simulink model "TractorTrailer6DOF"  (R2024b)
settings: Solver=ode23tb  StartTime=0.0  StopTime=50  MaxStep=1.0  RelTol=1e-1  AbsTol=1e-5
model mask{initialTractorPosition=[0 0 0], initialTractorVelocity=[0 0 0], initialTractorOrientation=[0 0 0], initialTractorRotationRates=[0 0 0], initialTrailerPosition=[0 0 0], initialTrailerVelocity=[0 0 0], initialTrailerOrientation=[0 0 0], initialTrailerRotationRates=[0 0 0]}
  mask prompts: initialTractorPosition "Initial Tractor Position:"; initialTractorVelocity "Initial Tractor Velocity:"; initialTractorOrientation "Initial Tractor Orientation:"; initialTractorRotationRates "Initial Tractor Rotation Rates:"; initialTrailerPosition "Initial Trailer Position:"; initialTrailerVelocity "Initial Trailer Velocity:"; initialTrailerOrientation "Initial Trailer Orientation:"; initialTrailerRotationRates "Initial Trailer Rotation Rates:"
model workspace (MAT data in the model file):
  initialTractorOrientation = Simulink.Parameter
  initialTractorOrientation.Value = [0 0 0]
  initialTractorOrientation.Complexity = 'real'
  initialTractorOrientation.Dimensions = [1 3]
  initialTractorOrientation.DataType = 'auto'
  initialTractorPosition = Simulink.Parameter
  initialTractorPosition.Value = [0 0 0]
  initialTractorPosition.Complexity = 'real'
  initialTractorPosition.Dimensions = [1 3]
  initialTractorPosition.DataType = 'auto'
  initialTractorRotationRates = Simulink.Parameter
  initialTractorRotationRates.Value = [0 0 0]
  initialTractorRotationRates.Complexity = 'real'
  initialTractorRotationRates.Dimensions = [1 3]
  initialTractorRotationRates.DataType = 'auto'
  initialTractorVelocity = Simulink.Parameter
  initialTractorVelocity.Value = [0 0 0]
  initialTractorVelocity.Complexity = 'real'
  initialTractorVelocity.Dimensions = [1 3]
  initialTractorVelocity.DataType = 'auto'
  initialTrailerOrientation = Simulink.Parameter
  initialTrailerOrientation.Value = [0 0 0]
  initialTrailerOrientation.Complexity = 'real'
  initialTrailerOrientation.Dimensions = [1 3]
  initialTrailerOrientation.DataType = 'auto'
  initialTrailerPosition = Simulink.Parameter
  initialTrailerPosition.Value = [0 0 0]
  initialTrailerPosition.Complexity = 'real'
  initialTrailerPosition.Dimensions = [1 3]
  initialTrailerPosition.DataType = 'auto'
  initialTrailerRotationRates = Simulink.Parameter
  initialTrailerRotationRates.Value = [0 0 0]
  initialTrailerRotationRates.Complexity = 'real'
  initialTrailerRotationRates.Dimensions = [1 3]
  initialTrailerRotationRates.DataType = 'auto'
  initialTrailerVelocity = Simulink.Parameter
  initialTrailerVelocity.Value = [0 0 0]
  initialTrailerVelocity.Complexity = 'real'
  initialTrailerVelocity.Dimensions = [1 3]
  initialTrailerVelocity.DataType = 'auto'
undefined symbols (not defined in the file): hitch, tractor, trailer
libraries: autolibutils x7, sharedtransform x4, vehdynlibtire x4, vehdynlibeom x2, vehdynlibsuspension x2, vehdynlibtirecommon x2, simulink x1
(part 1 of 4)
settings Model: SimulationMode=accelerator  ParameterArgumentNames=initialTractorOrientation,initialTractorPosition,initialTractorRotationRates,initialTractorVelocity,initialTrailerOrientation,initialTrailerPosition,initialTrailerRotationRates,initialTrailerVelocity  Creator=The MathWorks, Inc.  LastModifiedBy=rsuresh
settings SolverCC: DateTimeAtSimulationTimeZero=[]  SolverJacobianMethodControl=FullPerturbation  ZeroCrossAlgorithm=Adaptive  DecoupledContinuousIntegration=on  MinimalZcImpactIntegration=on
settings DataIOCC: ReturnWorkspaceOutputsName=tp280c6351_3b58_4b1a_80b9_cf8454703752
settings OptimizationCC: ReuseModelBlockBuffer=off
settings DebuggingCC: IgnoredZcDiagnostic=none
settings RTWCC: GPUComputeCapability=3.5

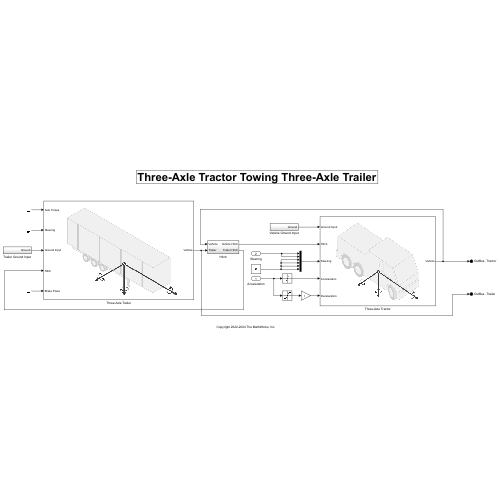
[thumbnail: Simulink's stored preview of the top-level diagram]
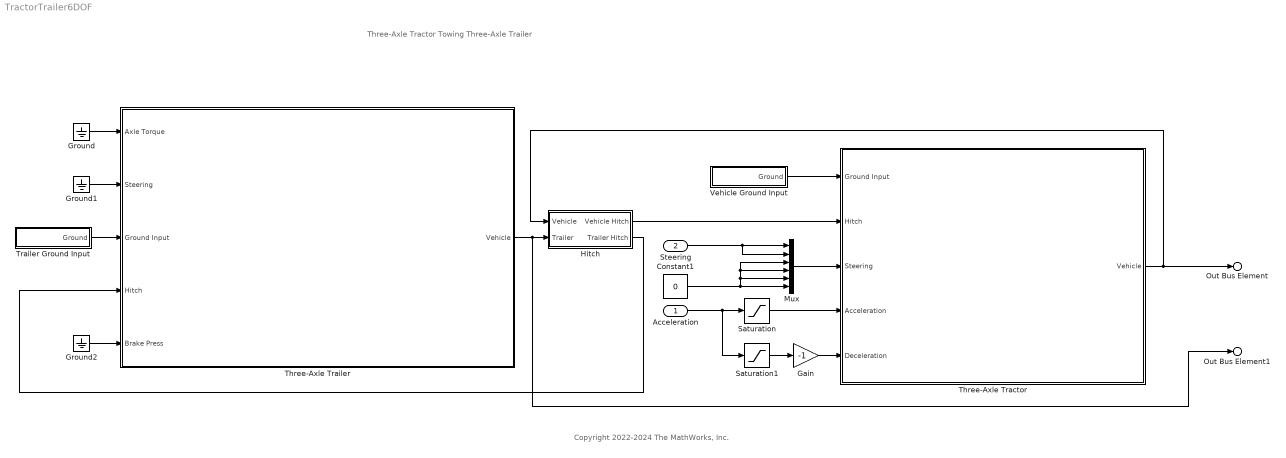
== system TractorTrailer6DOF ==
  note: Copyright 2022-2024 The MathWorks, Inc.
  note: Three-Axle Tractor Towing Three-Axle Trailer
  Acceleration : Inport
  Steering : Inport  Port=2
  Constant1 : Constant  Value=0
  Gain : Gain  Gain=-1
  Ground : Ground
  Ground1 : Ground
  Ground2 : Ground
  Hitch : Subsystem
  Mux : Mux  Inputs=6
  Saturation : Saturate  UpperLimit=3  LowerLimit=0  ZeroCross=off
  Saturation1 : Saturate  UpperLimit=0  LowerLimit=-9.8  ZeroCross=off
  Three-Axle Tractor : Subsystem
      mask Display: image('6dof3axletractor.png');
  Three-Axle Trailer : Subsystem
      mask Display: image('6dof3axletrailer.png');
  Trailer Ground Input : Subsystem  VariantControl=0
  Vehicle Ground Input : Subsystem  VariantControl=0
  Out Bus Element : Outport  PortName=OutBus  Element=Tractor
  Out Bus Element1 : Outport  PortName=OutBus  Element=Trailer
  wires:
  Ground2/1 -> Three-Axle Trailer/5(Brake Press)
  Gain/1 -> Three-Axle Tractor/5(Deceleration)
  Trailer Ground Input/1(Ground) -> Three-Axle Trailer/3(Ground Input)
  Ground/1 -> Three-Axle Trailer/1(Axle Torque)
  Vehicle Ground Input/1(Ground) -> Three-Axle Tractor/1(Ground Input)
  Ground1/1 -> Three-Axle Trailer/2(Steering)
  Hitch/2(Trailer Hitch) -> Three-Axle Trailer/4(Hitch)
  Mux/1 -> Three-Axle Tractor/3(Steering)
  Saturation1/1 -> Gain/1
  Saturation/1 -> Three-Axle Tractor/4(Acceleration)
  Hitch/1(Vehicle Hitch) -> Three-Axle Tractor/2(Hitch)
  Constant1/1 -> Mux/3, Mux/4, Mux/5, Mux/6
  Three-Axle Tractor/1(Vehicle) -> Out Bus Element/1, Hitch/1(Vehicle)
  Three-Axle Trailer/1(Vehicle) -> Out Bus Element1/1, Hitch/2(Trailer)
  Steering/1 -> Mux/2, Mux/1
  Acceleration/1 -> Saturation/1, Saturation1/1

== system TractorTrailer6DOF/Hitch ==
  Vehicle : Inport
  Trailer : Inport  Port=2
  Bus Selector : BusSelector  OutputSignals=Vehicle.InertFrm.Hitch.Disp.X,Vehicle.InertFrm.Hitch.Disp.Y,Vehicle.InertFrm.Hitch.Disp.Z,Vehicle.InertFrm.Hitch.Vel.Xdot,Vehicle.InertFrm.Hitch.Vel.Ydot,Vehicle.InertFrm.Hitch.Vel.Zdot,Vehicle.InertFrm.Cg.Ang.psi
  Bus Selector1 : BusSelector  OutputSignals=Vehicle.InertFrm.HitchF.Disp.X,Vehicle.InertFrm.HitchF.Disp.Y,Vehicle.InertFrm.HitchF.Disp.Z,Vehicle.InertFrm.HitchF.Vel.Xdot,Vehicle.InertFrm.HitchF.Vel.Ydot,Vehicle.InertFrm.HitchF.Vel.Zdot,Vehicle.InertFrm.Cg.Ang.psi
  Mux : Mux  Inputs=6
  Mux1 : Mux  Inputs=6
  Subsystem3 : Subsystem
  Vehicle Hitch : Outport
  Trailer Hitch : Outport  Port=2
  wires:
  Bus Selector1/5 -> Subsystem3/12(Trailer Ydot)  "<Ydot>"
  Subsystem3/5(Vehicle Mhy) -> Mux1/5
  Bus Selector/3 -> Subsystem3/3(Vehicle Z)  "<Z>"
  Subsystem3/12(Trailer Mhz) -> Mux/6
  Subsystem3/4(Vehicle Mhx) -> Mux1/4
  Subsystem3/10(Trailer Mhx) -> Mux/4
  Bus Selector/4 -> Subsystem3/4(Vehicle Xdot)  "<Xdot>"
  Subsystem3/11(Trailer Mhy) -> Mux/5
  Subsystem3/7(Trailer Fx) -> Mux/1
  Bus Selector1/1 -> Subsystem3/8(Trailer X)  "<X>"
  Bus Selector/5 -> Subsystem3/5(Vehicle Ydot)  "<Ydot>"
  Trailer/1 -> Bus Selector1/1
  Bus Selector1/4 -> Subsystem3/11(Trailer Xdot)  "<Xdot>"
  Subsystem3/6(Vehicle Mhz) -> Mux1/6
  Subsystem3/2(Vehicle Fy) -> Mux1/2
  Bus Selector/2 -> Subsystem3/2(Vehicle Y)  "<Y>"
  Bus Selector1/2 -> Subsystem3/9(Trailer Y)  "<Y>"
  Bus Selector1/6 -> Subsystem3/13(Trailer Zdot)  "<Zdot>"
  Subsystem3/1(Vehicle Fx) -> Mux1/1
  Bus Selector1/3 -> Subsystem3/10(Trailer Z)  "<Z>"
  Bus Selector/1 -> Subsystem3/1(Vehicle X)  "<X>"
  Subsystem3/8(Trailer Fy) -> Mux/2
  Bus Selector1/7 -> Subsystem3/14(Trailer psi)  "<psi>"
  Subsystem3/9(Trailer Fz) -> Mux/3
  Bus Selector/7 -> Subsystem3/7(Vehicle psi)  "<psi>"
  Mux/1 -> Trailer Hitch/1
  Bus Selector/6 -> Subsystem3/6(Vehicle Zdot)  "<Zdot>"
  Subsystem3/3(Vehicle Fz) -> Mux1/3
  Vehicle/1 -> Bus Selector/1
  Mux1/1 -> Vehicle Hitch/1

== system TractorTrailer6DOF/Three-Axle Tractor ==
  Ground Input : Inport
  Hitch : Inport  Port=2
  Steering : Inport  Port=3
  Acceleration : Inport  Port=4
  Deceleration : Inport  Port=5
  Brake System : Subsystem
  Brakes : BusCreator  Inputs=1
  Bus Creator : BusCreator  Inputs=4
  Bus Selector : BusSelector  OutputSignals=z,mu
  Subsystem1 : Subsystem
  Vehicle Body : Subsystem
  Vehicle Suspension : Subsystem
  Wheels and Tires : Subsystem
  Vehicle : Outport
  wires:
  Bus Selector/1 -> Wheels and Tires/4(Ground Input)  "<z>"
  Hitch/1 -> Vehicle Body/2(Hitch)
  Vehicle Suspension/1(Suspension) -> Wheels and Tires/1(Suspension), Bus Creator/2, Vehicle Body/1(Suspension)  "Suspension"
  Vehicle Body/1(Vehicle) -> Bus Creator/1, Vehicle Suspension/3(Vehicle), Brake System/2(Vehicle)  "Vehicle"
  Wheels and Tires/1(Wheels) -> Vehicle Suspension/2(Wheels), Bus Creator/3  "Wheels"
  Bus Selector/2 -> Wheels and Tires/5(Friction)  "<mu>"
  Steering/1 -> Vehicle Suspension/1(Steering)
  Ground Input/1 -> Bus Selector/1
  Bus Creator/1 -> Vehicle/1
  Brake System/1(Brake Press) -> Brakes/1, Wheels and Tires/3(Brake Press)  "Pressure"
  Deceleration/1 -> Brake System/1(Deceleration)
  Brakes/1 -> Bus Creator/4  "Brakes"
  Subsystem1/1(TAxles) -> Wheels and Tires/2(Axle Torque)
  Wheels and Tires/2(AxlPwr) -> [AxlPwr]
  Wheels and Tires/3(Omega) -> [Omega]
  Acceleration/1 -> Subsystem1/1(Acceleration)
  [AxlPwr] -> Subsystem1/2(AxlPwr)
  [Omega] -> Subsystem1/3(Omega)

== system TractorTrailer6DOF/Three-Axle Trailer ==
  Axle Torque : Inport
  Steering : Inport  Port=2
  Ground Input : Inport  Port=3
  Hitch : Inport  Port=4
  Brake Press : Inport  Port=5
  Brakes : BusCreator  Inputs=1
  Bus Creator : BusCreator  Inputs=4
  Bus Selector : BusSelector  OutputSignals=z,mu
  Trailer Suspension : Subsystem
  Vehicle Body : Subsystem
  Wheels and Tires : Subsystem
  Vehicle : Outport
  wires:
  Bus Creator/1 -> Vehicle/1
  Ground Input/1 -> Bus Selector/1
  Steering/1 -> Trailer Suspension/1(Steering)
  Axle Torque/1 -> Wheels and Tires/2(Axle Torque)
  Bus Selector/2 -> Wheels and Tires/5(Friction)  "<mu>"
  Wheels and Tires/1(Wheels) -> Trailer Suspension/2(Wheels), Bus Creator/3  "Wheels"
  Vehicle Body/1(Vehicle) -> Bus Creator/1, Trailer Suspension/3(Vehicle)  "Vehicle"
  Trailer Suspension/1(Suspension) -> Wheels and Tires/1(Suspension), Bus Creator/2, Vehicle Body/1(Suspension)  "Suspension"
  Hitch/1 -> Vehicle Body/2(Hitch)
  Bus Selector/1 -> Wheels and Tires/4(Ground Input)  "<z>"
  Brakes/1 -> Bus Creator/4  "Brakes"
  Brake Press/1 -> Wheels and Tires/3(Brake Press), Brakes/1  "Pressure"

== system TractorTrailer6DOF/Trailer Ground Input ==
  Bus Creator : BusCreator  Inputs=6
  Bus Creator2 : BusCreator  Inputs=6
  Bus Creator3 : BusCreator  Inputs=2
  Constant1 : Constant  Value=zeros(6,1)
  Demux : Demux  Outputs=6
  Demux1 : Demux  Outputs=6
  Friction : Constant  Value=ones(6,1).*1.0
  Signal Specification : SignalSpecification  Unit=m
  Signal Specification1 : SignalSpecification  Unit=1
  Ground : Outport  VectorParamsAs1DForOutWhenUnconnected=off
  wires:
  Constant1/1 -> Signal Specification/1
  Signal Specification/1 -> Demux/1
  Demux/6 -> Bus Creator/6  "G_RR_z"
  Demux/1 -> Bus Creator/1  "G_FL_z"
  Demux/5 -> Bus Creator/5  "G_RL_z"
  Demux/2 -> Bus Creator/2  "G_FR_z"
  Bus Creator/1 -> Bus Creator3/1  "z"
  Demux1/5 -> Bus Creator2/5  "mu_RL"
  Demux1/6 -> Bus Creator2/6  "mu_RR"
  Demux1/1 -> Bus Creator2/1  "mu_FL"
  Demux1/2 -> Bus Creator2/2  "mu_FR"
  Bus Creator2/1 -> Bus Creator3/2  "mu"
  Friction/1 -> Signal Specification1/1
  Signal Specification1/1 -> Demux1/1
  Bus Creator3/1 -> Ground/1
  Demux/3 -> Bus Creator/3  "G_ML_z"
  Demux/4 -> Bus Creator/4  "G_MR_z"
  Demux1/3 -> Bus Creator2/3  "mu_ML"
  Demux1/4 -> Bus Creator2/4  "mu_MR"

== system TractorTrailer6DOF/Vehicle Ground Input ==
  Bus Creator : BusCreator  Inputs=6
  Bus Creator2 : BusCreator  Inputs=6
  Bus Creator3 : BusCreator  Inputs=2
  Constant1 : Constant  Value=zeros(6,1)
  Demux : Demux  Outputs=6
  Demux1 : Demux  Outputs=6
  Friction : Constant  Value=ones(6,1).*1.0
  Signal Specification : SignalSpecification  Unit=m
  Signal Specification1 : SignalSpecification  Unit=1
  Ground : Outport  VectorParamsAs1DForOutWhenUnconnected=off
  wires:
  Demux1/4 -> Bus Creator2/4  "mu_MR"
  Demux1/3 -> Bus Creator2/3  "mu_ML"
  Demux/4 -> Bus Creator/4  "G_MR_z"
  Demux/3 -> Bus Creator/3  "G_ML_z"
  Bus Creator3/1 -> Ground/1
  Signal Specification1/1 -> Demux1/1
  Friction/1 -> Signal Specification1/1
  Bus Creator2/1 -> Bus Creator3/2  "mu"
  Demux1/2 -> Bus Creator2/2  "mu_FR"
  Demux1/1 -> Bus Creator2/1  "mu_FL"
  Demux1/6 -> Bus Creator2/6  "mu_RR"
  Demux1/5 -> Bus Creator2/5  "mu_RL"
  Bus Creator/1 -> Bus Creator3/1  "z"
  Demux/2 -> Bus Creator/2  "G_FR_z"
  Demux/5 -> Bus Creator/5  "G_RL_z"
  Demux/1 -> Bus Creator/1  "G_FL_z"
  Demux/6 -> Bus Creator/6  "G_RR_z"
  Signal Specification/1 -> Demux/1
  Constant1/1 -> Signal Specification/1

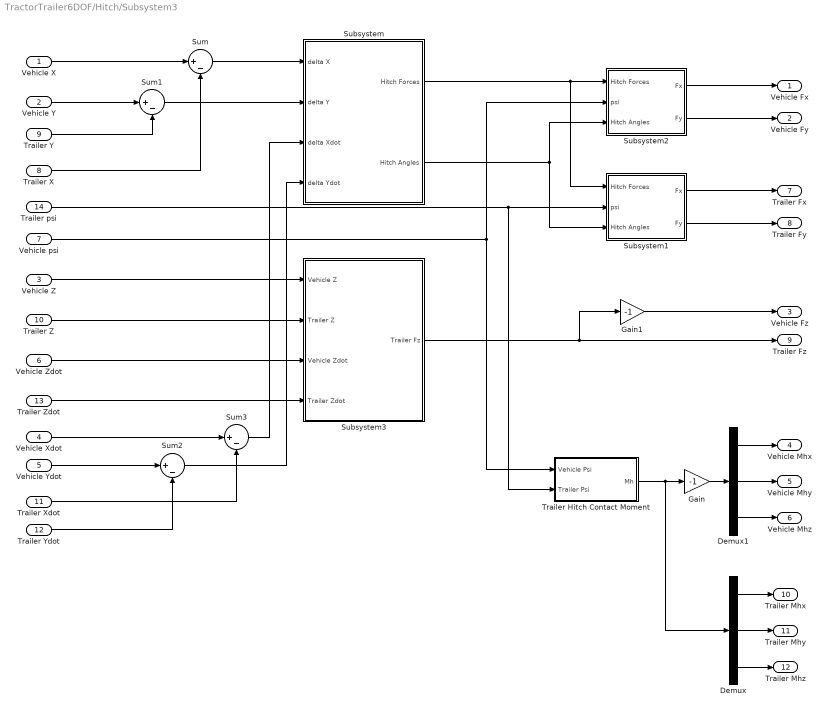
== system TractorTrailer6DOF/Hitch/Subsystem3 ==
  Vehicle X : Inport
  Vehicle Y : Inport  Port=2
  Vehicle Z : Inport  Port=3
  Vehicle Xdot : Inport  Port=4
  Vehicle Ydot : Inport  Port=5
  Vehicle Zdot : Inport  Port=6
  Vehicle psi : Inport  Port=7
  Trailer X : Inport  Port=8
  Trailer Y : Inport  Port=9
  Trailer Z : Inport  Port=10
  Trailer Xdot : Inport  Port=11
  Trailer Ydot : Inport  Port=12
  Trailer Zdot : Inport  Port=13
  Trailer psi : Inport  Port=14
  Demux : Demux  Outputs=3
  Demux1 : Demux  Outputs=3
  Gain : Gain  Gain=-1
  Gain1 : Gain  Gain=-1
  Subsystem : Subsystem
  Subsystem1 : Subsystem
  Subsystem2 : Subsystem
  Subsystem3 : Subsystem
  Sum{,1..3} (4 alike) : Sum  Inputs=|+-
  Trailer Hitch Contact Moment : Subsystem
  Vehicle Fx : Outport
  Vehicle Fy : Outport  Port=2
  Vehicle Fz : Outport  Port=3
  Vehicle Mhx : Outport  Port=4
  Vehicle Mhy : Outport  Port=5
  Vehicle Mhz : Outport  Port=6
  Trailer Fx : Outport  Port=7
  Trailer Fy : Outport  Port=8
  Trailer Fz : Outport  Port=9
  Trailer Mhx : Outport  Port=10
  Trailer Mhy : Outport  Port=11
  Trailer Mhz : Outport  Port=12
  wires:
  Subsystem/1(Hitch Forces) -> Subsystem2/1(Hitch Forces), Subsystem1/1(Hitch Forces)
  Sum/1 -> Subsystem/1(delta X)
  Sum1/1 -> Subsystem/2(delta Y)
  Vehicle X/1 -> Sum/1
  Trailer Y/1 -> Sum1/2
  Trailer X/1 -> Sum/2
  Vehicle Y/1 -> Sum1/1
  Trailer psi/1 -> Trailer Hitch Contact Moment/2(Trailer Psi), Subsystem1/2(psi)
  Vehicle psi/1 -> Subsystem2/2(psi), Trailer Hitch Contact Moment/1(Vehicle Psi)
  Subsystem/2(Hitch Angles) -> Subsystem2/3(Hitch Angles), Subsystem1/3(Hitch Angles)
  Subsystem3/1(Trailer Fz) -> Gain1/1, Trailer Fz/1
  Subsystem2/1(Fx) -> Vehicle Fx/1
  Subsystem2/2(Fy) -> Vehicle Fy/1
  Subsystem1/1(Fx) -> Trailer Fx/1
  Subsystem1/2(Fy) -> Trailer Fy/1
  Vehicle Z/1 -> Subsystem3/1(Vehicle Z)
  Trailer Z/1 -> Subsystem3/2(Trailer Z)
  Gain1/1 -> Vehicle Fz/1
  Vehicle Zdot/1 -> Subsystem3/3(Vehicle Zdot)
  Trailer Zdot/1 -> Subsystem3/4(Trailer Zdot)
  Trailer Ydot/1 -> Sum2/2
  Vehicle Xdot/1 -> Sum3/1
  Vehicle Ydot/1 -> Sum2/1
  Trailer Xdot/1 -> Sum3/2
  Sum2/1 -> Subsystem/4(delta Ydot)
  Sum3/1 -> Subsystem/3(delta Xdot)
  Demux/1 -> Trailer Mhx/1
  Demux1/3 -> Vehicle Mhz/1
  Demux/2 -> Trailer Mhy/1
  Demux1/2 -> Vehicle Mhy/1
  Trailer Hitch Contact Moment/1(Mh) -> Demux/1, Gain/1
  Demux1/1 -> Vehicle Mhx/1
  Demux/3 -> Trailer Mhz/1
  Gain/1 -> Demux1/1

== system TractorTrailer6DOF/Three-Axle Tractor/Brake System ==
  Deceleration : Inport
  Vehicle : Inport  Port=2
  Bus Selector : BusSelector  OutputSignals=BdyFrm.Cg.Vel.xdot
  Constant : Constant  Value=0
  Hydraulics : autolibutils/Cont LPF  wc=30*pi*2  AbsoluteTolerance=auto  aMode=2
  Mux : Mux  Inputs=6
  Pressure : Gain  Gain=2e5
  Pressure1 : Gain  Gain=1e6
  Saturation1 : Saturate  UpperLimit=inf  LowerLimit=0  ZeroCross=off
  Signal Specification : SignalSpecification  Unit=Pa
  Switch : Switch  Criteria=u2 > Threshold  Threshold=0.1  ZeroCross=off  SaturateOnIntegerOverflow=off  InputSameDT=off
  Brake Press : Outport  PortDimensions=6  VectorParamsAs1DForOutWhenUnconnected=off
  wires:
  Signal Specification/1 -> Brake Press/1
  Mux/1 -> Signal Specification/1
  Saturation1/1 -> Hydraulics/1
  Hydraulics/1 -> Pressure1/1, Pressure/1
  Pressure/1 -> Mux/2, Mux/1
  Vehicle/1 -> Bus Selector/1
  Switch/1 -> Saturation1/1
  Deceleration/1 -> Switch/1
  Bus Selector/1 -> Switch/2  "<xdot>"
  Constant/1 -> Switch/3
  Pressure1/1 -> Mux/6, Mux/4, Mux/3, Mux/5

== system TractorTrailer6DOF/Three-Axle Tractor/Subsystem1 ==
  Acceleration : Inport
  AxlPwr : Inport  Port=2
  Omega : Inport  Port=3
  Constant : Constant
  Driveline : Subsystem  Variant=on  VariantControlMode=label  VariantControl=Variant1  LabelModeActiveChoice=0
  Powertrain : Subsystem
  TAxles : Outport
  wires:
  Powertrain/1(AxlTrq) -> Driveline/1(TPowertrain)
  Acceleration/1 -> Powertrain/1(Acc)
  Omega/1 -> Powertrain/3(Omega)
  AxlPwr/1 -> Powertrain/2(AxlPwr)
  Driveline/1(TAxles) -> TAxles/1
  Constant/1 -> Driveline/2(Gear)

== system TractorTrailer6DOF/Three-Axle Tractor/Vehicle Body ==
  Suspension : Inport
  Hitch : Inport  Port=2
  Bus Selector3 : BusSelector  OutputSignals=Veh.F,Veh.M
  Constant : Constant  Value=zeros(3,1)
  Ground : Ground
  Ground1 : Ground
  Selector6 : Selector  InputPortWidth=6  IndexOptions=Index vector (dialog)  Indices=[1 2 3]  OutputSizes=1
  Selector7 : Selector  InputPortWidth=6  IndexOptions=Index vector (dialog)  Indices=[4 5 6]  OutputSizes=1
  Terminator{6..11} (6 alike) : Terminator
  Vehicle Body 6DOF Three Axles : vehdynlibeom/Vehicle Body 6DOF Three Axles  extPos=on  extVel=on  extEuler=on  extRotRate=on  htchFMode=on  htchMMode=on  m=tractor.Mass  a=tractor.FrontAxlePositionfromCG  b=tractor.MiddleAxlePositionFromCG  c=tractor.RearAxlePositionfromCG  d=0  h=tractor.HeightCG  dh=tractor.HitchDistance  hl=0  hh=tractor.HitchHeight  Xe_o=initialTractorPosition  xbdot_o=initialTractorVelocity  eul_o=initialTractorOrientation  p_o=initialTractorRotationRates  Iveh=[tractor.RollMomentInertia 0 0; 0 tractor.PitchMomentInertia 0; 0 0 tractor.YawMomentInertia]  w=tractor.TrackWidth.*[1 1 1]  z1m=0  z1R=[-.25,.125,.15]  z1I=[1.4,-.2,.1;-.2,1.4,.1;.1,.1,2.25].*0  z2m=0  z2R=[1.4,0,.8]  z2I=[1.4,-.2,.1;-.2,1.4,.1;.1,.1,2.25].*0  z3m=0  z3R=[.75,-.5,.4]  z3I=[5,-.1,-2;-2,9,.1;-.1,.1,6].*0  z4m=0  z4R=[.75,.5,.4]  z4I=[5,-.1,-2;-2,9,.1;-.1,.1,6].*0  z5m=0  z5R=[1.25,-.5,.4]  z5I=[5,-.1,-2;-2,9,.1;-.1,.1,6].*0  z6m=0  z6R=[1.25,-.5,.4]  z6I=[5,-.1,-2;-2,9,.1;-.1,.1,6].*0  z7m=0  z7R=[2,0,.25]  z7I=[1.4,-.2,.1;-.2,1.4,.1;.1,.1,2.25].*0  Af=tractor.FrontalArea  Cd=.3  Cl=.1  Cpm=.1  beta_w=[0:0.01:0.3]  Cs=[0:0.03:0.9]  Cym=[0:0.01:0.3]  Pabs=101325  extTamb=off  Tair=273  g=9.81  xdot_tol=.1  longOff=0  latOff=0  vertOff=0.0112  wrapAng=off  aMode=2
  Vehicle : Outport
  wires:
  Suspension/1 -> Bus Selector3/1
  Selector6/1 -> Vehicle Body 6DOF Three Axles/5
  Vehicle Body 6DOF Three Axles/2 -> Terminator6/1
  Hitch/1 -> Selector7/1, Selector6/1
  Vehicle Body 6DOF Three Axles/4 -> Terminator8/1
  Ground/1 -> Vehicle Body 6DOF Three Axles/3
  Vehicle Body 6DOF Three Axles/6 -> Terminator10/1
  Selector7/1 -> Vehicle Body 6DOF Three Axles/6
  Constant/1 -> Vehicle Body 6DOF Three Axles/7
  Vehicle Body 6DOF Three Axles/1 -> Vehicle/1
  Vehicle Body 6DOF Three Axles/3 -> Terminator7/1
  Bus Selector3/2 -> Vehicle Body 6DOF Three Axles/2  "<M>"
  Bus Selector3/1 -> Vehicle Body 6DOF Three Axles/1  "<F>"
  Vehicle Body 6DOF Three Axles/7 -> Terminator11/1
  Ground1/1 -> Vehicle Body 6DOF Three Axles/4
  Vehicle Body 6DOF Three Axles/5 -> Terminator9/1

== system TractorTrailer6DOF/Three-Axle Tractor/Vehicle Suspension ==
  Steering : Inport
  Wheels : Inport  Port=2
  Vehicle : Inport  Port=3
  Bus Creator1 : BusCreator  Inputs=5
  Bus Creator2 : BusCreator  Inputs=2
  Bus Creator3 : BusCreator  Inputs=2
  Bus Creator4 : BusCreator  Inputs=6
  Bus Selector : BusSelector  OutputSignals=z,Re,zdot,Fx,Fy,M
  Bus Selector1 : BusSelector  OutputSignals=P,V
  Selector1 : Selector  NumberOfDimensions=2  InputPortWidth=3  IndexOptions=Index vector (dialog),Select all  Indices=1,1  OutputSizes=1,1
  Selector2 : Selector  NumberOfDimensions=2  InputPortWidth=3  IndexOptions=Index vector (dialog),Select all  Indices=2,1  OutputSizes=1,1
  Solid Axle Suspension - Coil Spring : vehdynlibsuspension/Solid Axle Suspension - Coil Spring  NumAxl=3  NumWhlsByAxl=[2 2 2]  StrgEnByAxl=[1 1 1]  WhlNumVec="[1  2  1  2  1  2]"  AxleNumVec="[1  1  2  2  3  3]"  SuspTypesByAxle="[1  1  1]"  SuspImage=suspsacoil.png  AxlIxx=450  AxlM=500  TrackCoords=[zeros(1,6);tractor.TrackWidth*[1 -1 1 -1 1 -1]/2;zeros(1,6)]  SuspCoords=[zeros(1,6);tractor.TrackWidth*[1 -1 1 -1 1 -1]/2;zeros(1,6)]  KzWhlAxl=kzWhlAxl  F0zWhlAxl=f0zWhlAxl  CzWhlAxl=czWhlAxl  IdealSuspEn=on  IdealSuspAxles="[1  2  3]"  Kz=tractor.Kz  F0z=tractor.F0z  Cz=tractor.Cz  Hmax=hMax  Toe=0  RollStrgSlp=0  ToeStrgSlp=0  Caster=0  CasterHslp=0  CasterStrgSlp=0  Camber=0  CamberHslp=0  CamberStrgSlp=0  StrgHgtSlp=0.1432  MappedSuspEn=off  MappedSuspAxles="[1  2]"  f_susp_axl_bp=[1 2]  f_susp_dz_bp=[-0.15 -0.14 -0.13 -0.12 -0.11 -0.10 -0.09 -0.08 -0.07 -0.06 -0.05 -0.04 -0.03 -0.02 -0.01 0.00 0.01 0.02 0.03 0.04 0.05 0.06 0.07 0.08 0.09 0.10 0.11 0.12 0.13 0.14 0.15]  f_susp_dzdot_bp=[-0.15 -0.14 -0.13 -0.12 -0.11 -0.10 -0.09 -0.08 -0.07 -0.06 -0.05 -0.04 -0.03 -0.02 -0.01 0.00 0.01 0.02 0.03 0.04 0.05 0.06 0.07 0.08 0.09 0.10 0.11 0.12 0.13 0.14 0.15]  f_susp_fmz=zeros(31,31,61,2,4)  f_susp_geom=zeros(31,61,2,3)  f_susp_strgdelta_bp=[-30,-29,-28,-27,-26,-25,-24,-23,-22,-21,-20,-19,-18,-17,-16,-15,-14,-13,-12,-11,-10,-9,-8,-7,-6,-5,-4,-3,-2,-1,0,1,2,3,4,5,6,7,8,9,10,11,12,13,14,15,16,17,18,19,20,21,22,23,24,25,26,27,28,29,30]
  Steer Rate Adapter : Subsystem
  Steering Adapter : Subsystem
  Terminator1 : Terminator
  Terminator6 : Terminator
  Vehicle Adapter : Subsystem
  Wheel  Adapter : Subsystem
  Suspension : Outport
  wires:
  Wheel  Adapter/6(Re) -> Bus Creator4/6
  Bus Selector1/1 -> Solid Axle Suspension - Coil Spring/7  "<P>"
  Bus Selector/6 -> Solid Axle Suspension - Coil Spring/6  "<M>"
  Bus Selector/1 -> Solid Axle Suspension - Coil Spring/1  "<z>"
  Bus Selector/5 -> Solid Axle Suspension - Coil Spring/5  "<Fy>"
  Wheel  Adapter/1(WhlFx) -> Bus Creator4/1  "Fx"
  Bus Selector/4 -> Solid Axle Suspension - Coil Spring/4  "<Fx>"
  Wheel  Adapter/4(zdot) -> Bus Creator4/4
  Wheel  Adapter/2(WhlFy) -> Bus Creator4/2  "Fy"
  Solid Axle Suspension - Coil Spring/1 -> Terminator6/1
  Vehicle Adapter/1(VehSusp) -> Bus Selector1/1
  Bus Creator4/1 -> Bus Selector/1
  Bus Selector1/2 -> Solid Axle Suspension - Coil Spring/8  "<V>"
  Steering/1 -> Steering Adapter/1(Steer)
  Bus Selector/3 -> Solid Axle Suspension - Coil Spring/3  "<zdot>"
  Wheel  Adapter/3(z) -> Bus Creator4/3
  Wheel  Adapter/5(M) -> Bus Creator4/5
  Bus Selector/2 -> Solid Axle Suspension - Coil Spring/2  "<Re>"
  Vehicle Adapter/2(VehVBody) -> Selector1/1, Selector2/1
  Wheels/1 -> Wheel  Adapter/1(Wheels)
  Steering Adapter/1(StrgAng) -> Solid Axle Suspension - Coil Spring/9
  Vehicle/1 -> Vehicle Adapter/1(Veh), Steer Rate Adapter/1(Veh)
  Bus Creator3/1 -> Suspension/1
  Selector2/1 -> Bus Creator1/3  "ydot"
  Bus Creator2/1 -> Bus Creator3/1  "Veh"
  Solid Axle Suspension - Coil Spring/3 -> Bus Creator2/2  "M"
  Selector1/1 -> Bus Creator1/2  "xdot"
  Solid Axle Suspension - Coil Spring/6 -> Bus Creator1/4  "Ang"
  Bus Creator1/1 -> Bus Creator3/2  "Whl"
  Steer Rate Adapter/1(AngVel) -> Bus Creator1/5
  Solid Axle Suspension - Coil Spring/2 -> Bus Creator2/1  "F"
  Solid Axle Suspension - Coil Spring/4 -> Bus Creator1/1  "F"
  Solid Axle Suspension - Coil Spring/5 -> Terminator1/1

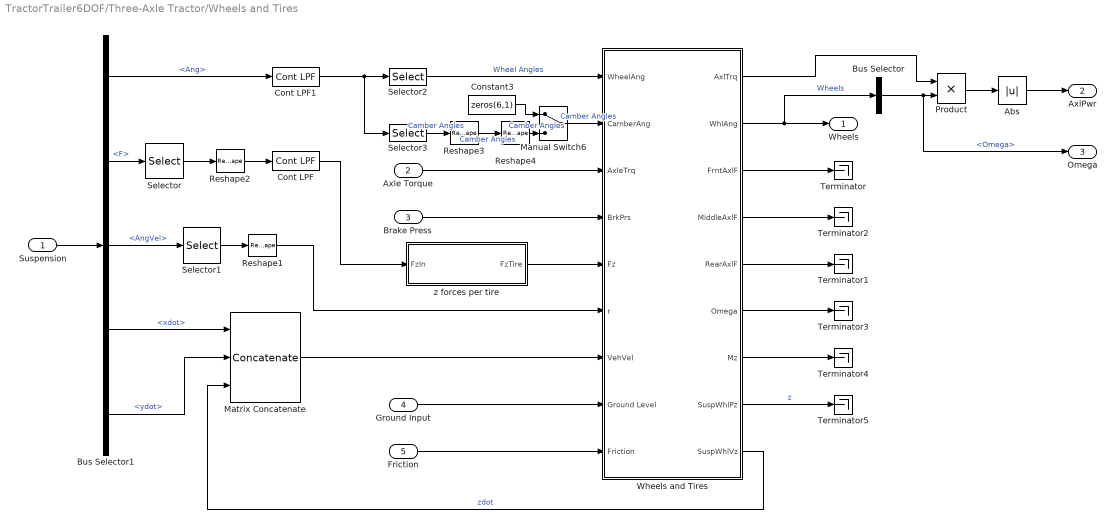
== system TractorTrailer6DOF/Three-Axle Tractor/Wheels and Tires ==
  Suspension : Inport
  Axle Torque : Inport  Port=2
  Brake Press : Inport  Port=3  Unit=Pa
  Ground Input : Inport  Port=4
  Friction : Inport  Port=5
  Abs : Abs  SaturateOnIntegerOverflow=off
  Bus Selector : BusSelector  OutputSignals=TireFrame.Omega
  Bus Selector1 : BusSelector  OutputSignals=Whl.Ang,Whl.F,Whl.AngVel,Whl.xdot,Whl.ydot
  Constant3 : Constant  Value=zeros(6,1)
  Cont LPF : autolibutils/Cont LPF  wc=100*2*pi  AbsoluteTolerance=auto  aMode=2
  Cont LPF1 : autolibutils/Cont LPF  wc=100*2*pi  AbsoluteTolerance=auto  aMode=2
  Manual Switch6 : ManualSwitch
  Matrix Concatenate : Concatenate  NumInputs=3  Mode=Multidimensional array
  Product : Product
  Reshape1 : Reshape
  Reshape2 : Reshape
  Reshape3 : Reshape  OutputDimensionality=Column vector (2-D)
  Reshape4 : Reshape
  Selector : Selector  NumberOfDimensions=2  InputPortWidth=3  IndexOptions=Index vector (dialog),Select all  Indices=[3],1  OutputSizes=1,1
  Selector1 : Selector  NumberOfDimensions=2  InputPortWidth=1  IndexOptions=Index vector (dialog),Select all  Indices=[3],1  OutputSizes=1,1
  Selector2 : Selector  NumberOfDimensions=2  InputPortWidth=3  IndexOptions=Index vector (dialog),Select all  Indices=3,1  OutputSizes=1,1
  Selector3 : Selector  NumberOfDimensions=2  InputPortWidth=3  IndexOptions=Index vector (dialog),Select all  Indices=1,1  OutputSizes=1,1
  Terminator{,1..5} (6 alike) : Terminator
  Wheels and Tires : Subsystem  VariantControl=0
  z forces per tire : Subsystem
  Wheels : Outport  VectorParamsAs1DForOutWhenUnconnected=off
  AxlPwr : Outport  Port=2
  Omega : Outport  Port=3
  wires:
  Wheels and Tires/2(WhlAng) -> Bus Selector/1, Wheels/1  "Wheels"
  Bus Selector1/2 -> Selector/1  "<F>"
  Wheels and Tires/3(FrntAxlF) -> Terminator/1
  Wheels and Tires/5(RearAxlF) -> Terminator1/1
  Wheels and Tires/6(Omega) -> Terminator3/1
  Wheels and Tires/7(Mz) -> Terminator4/1
  Selector1/1 -> Reshape1/1
  Matrix Concatenate/1 -> Wheels and Tires/7(VehVel)
  Axle Torque/1 -> Wheels and Tires/3(AxleTrq)
  Selector2/1 -> Wheels and Tires/1(WheelAng)  "Wheel Angles"
  Constant3/1 -> Manual Switch6/1
  Manual Switch6/1 -> Wheels and Tires/2(CamberAng)  "Camber Angles"
  Selector/1 -> Reshape2/1
  z forces per tire/1(FzTire) -> Wheels and Tires/5(Fz)
  Ground Input/1 -> Wheels and Tires/8(Ground Level)
  Wheels and Tires/9(SuspWhlVz) -> Matrix Concatenate/3  "zdot"
  Bus Selector1/1 -> Cont LPF1/1  "<Ang>"
  Selector3/1 -> Reshape3/1  "Camber Angles"
  Suspension/1 -> Bus Selector1/1
  Bus Selector1/4 -> Matrix Concatenate/1  "<xdot>"
  Bus Selector1/5 -> Matrix Concatenate/2  "<ydot>"
  Wheels and Tires/8(SuspWhlPz) -> Terminator5/1  "z"
  Reshape2/1 -> Cont LPF/1
  Bus Selector1/3 -> Selector1/1  "<AngVel>"
  Reshape1/1 -> Wheels and Tires/6(r)
  Brake Press/1 -> Wheels and Tires/4(BrkPrs)
  Friction/1 -> Wheels and Tires/9(Friction)
  Cont LPF1/1 -> Selector3/1, Selector2/1
  Wheels and Tires/4(MiddleAxlF) -> Terminator2/1
  Reshape3/1 -> Reshape4/1  "Camber Angles"
  Reshape4/1 -> Manual Switch6/2  "Camber Angles"
  Cont LPF/1 -> z forces per tire/1(FzIn)
  Bus Selector/1 -> Omega/1, Product/2  "<Omega>"
  Wheels and Tires/1(AxlTrq) -> Product/1
  Product/1 -> Abs/1
  Abs/1 -> AxlPwr/1

== system TractorTrailer6DOF/Three-Axle Trailer/Trailer Suspension ==
  Steering : Inport
  Wheels : Inport  Port=2
  Vehicle : Inport  Port=3
  Bus Creator1 : BusCreator  Inputs=5
  Bus Creator2 : BusCreator  Inputs=2
  Bus Creator3 : BusCreator  Inputs=2
  Bus Creator4 : BusCreator  Inputs=6
  Bus Selector : BusSelector  OutputSignals=z,Re,zdot,Fx,Fy,M
  Bus Selector1 : BusSelector  OutputSignals=P,V
  Selector1 : Selector  NumberOfDimensions=2  InputPortWidth=3  IndexOptions=Index vector (dialog),Select all  Indices=1,1  OutputSizes=1,1
  Selector2 : Selector  NumberOfDimensions=2  InputPortWidth=3  IndexOptions=Index vector (dialog),Select all  Indices=2,1  OutputSizes=1,1
  Solid Axle Suspension - Coil Spring : vehdynlibsuspension/Solid Axle Suspension - Coil Spring  NumAxl=3  NumWhlsByAxl=[2 2 2]  StrgEnByAxl=[1 1 1]  WhlNumVec="[1  2  1  2  1  2]"  AxleNumVec="[1  1  2  2  3  3]"  SuspTypesByAxle="[1  1  1]"  SuspImage=suspsacoil.png  AxlIxx=450  AxlM=500  TrackCoords=[zeros(1,6);trailer.TrackWidth*[1 -1 1 -1 1 -1]/2;zeros(1,6)]  SuspCoords=[zeros(1,6);trailer.TrackWidth*[1 -1 1 -1 1 -1]/2;zeros(1,6)]  KzWhlAxl=kzWhlAxl  F0zWhlAxl=f0zWhlAxl  CzWhlAxl=czWhlAxl  IdealSuspEn=on  IdealSuspAxles="[1  2  3]"  Kz=trailer.Kz  F0z=trailer.F0z  Cz=trailer.Cz(1)  Hmax=hMax  Toe=0  RollStrgSlp=0  ToeStrgSlp=0  Caster=0  CasterHslp=0  CasterStrgSlp=0  Camber=0  CamberHslp=0  CamberStrgSlp=0  StrgHgtSlp=0.1432  MappedSuspEn=off  MappedSuspAxles="[1  2]"  f_susp_axl_bp=[1 2]  f_susp_dz_bp=[-0.15 -0.14 -0.13 -0.12 -0.11 -0.10 -0.09 -0.08 -0.07 -0.06 -0.05 -0.04 -0.03 -0.02 -0.01 0.00 0.01 0.02 0.03 0.04 0.05 0.06 0.07 0.08 0.09 0.10 0.11 0.12 0.13 0.14 0.15]  f_susp_dzdot_bp=[-0.15 -0.14 -0.13 -0.12 -0.11 -0.10 -0.09 -0.08 -0.07 -0.06 -0.05 -0.04 -0.03 -0.02 -0.01 0.00 0.01 0.02 0.03 0.04 0.05 0.06 0.07 0.08 0.09 0.10 0.11 0.12 0.13 0.14 0.15]  f_susp_fmz=zeros(31,31,61,2,4)  f_susp_geom=zeros(31,61,2,3)  f_susp_strgdelta_bp=[-30,-29,-28,-27,-26,-25,-24,-23,-22,-21,-20,-19,-18,-17,-16,-15,-14,-13,-12,-11,-10,-9,-8,-7,-6,-5,-4,-3,-2,-1,0,1,2,3,4,5,6,7,8,9,10,11,12,13,14,15,16,17,18,19,20,21,22,23,24,25,26,27,28,29,30]
  Steer Rate Adapter : Subsystem
  Steering Adapter : Subsystem
  Terminator1 : Terminator
  Terminator6 : Terminator
  Vehicle Adapter : Subsystem
  Wheel  Adapter : Subsystem
  Suspension : Outport
  wires:
  Steer Rate Adapter/1(AngVel) -> Bus Creator1/5
  Bus Creator1/1 -> Bus Creator3/2  "Whl"
  Solid Axle Suspension - Coil Spring/6 -> Bus Creator1/4  "Ang"
  Selector1/1 -> Bus Creator1/2  "xdot"
  Solid Axle Suspension - Coil Spring/3 -> Bus Creator2/2  "M"
  Bus Creator2/1 -> Bus Creator3/1  "Veh"
  Selector2/1 -> Bus Creator1/3  "ydot"
  Bus Creator3/1 -> Suspension/1
  Vehicle/1 -> Steer Rate Adapter/1(Veh), Vehicle Adapter/1(Veh)
  Steering Adapter/1(StrgAng) -> Solid Axle Suspension - Coil Spring/9
  Wheels/1 -> Wheel  Adapter/1(Wheels)
  Vehicle Adapter/1(VehVBody) -> Selector1/1, Selector2/1
  Bus Selector/2 -> Solid Axle Suspension - Coil Spring/2  "<Re>"
  Wheel  Adapter/5(M) -> Bus Creator4/5
  Wheel  Adapter/3(z) -> Bus Creator4/3
  Bus Selector/3 -> Solid Axle Suspension - Coil Spring/3  "<zdot>"
  Steering/1 -> Steering Adapter/1(Steer)
  Bus Selector1/2 -> Solid Axle Suspension - Coil Spring/8  "<V>"
  Bus Creator4/1 -> Bus Selector/1
  Solid Axle Suspension - Coil Spring/1 -> Terminator6/1
  Wheel  Adapter/2(WhlFy) -> Bus Creator4/2  "Fy"
  Wheel  Adapter/4(zdot) -> Bus Creator4/4
  Bus Selector/4 -> Solid Axle Suspension - Coil Spring/4  "<Fx>"
  Wheel  Adapter/1(WhlFx) -> Bus Creator4/1  "Fx"
  Bus Selector/5 -> Solid Axle Suspension - Coil Spring/5  "<Fy>"
  Bus Selector/1 -> Solid Axle Suspension - Coil Spring/1  "<z>"
  Bus Selector/6 -> Solid Axle Suspension - Coil Spring/6  "<M>"
  Bus Selector1/1 -> Solid Axle Suspension - Coil Spring/7  "<P>"
  Wheel  Adapter/6(Re) -> Bus Creator4/6
  Solid Axle Suspension - Coil Spring/2 -> Bus Creator2/1  "F"
  Solid Axle Suspension - Coil Spring/4 -> Bus Creator1/1  "F"
  Solid Axle Suspension - Coil Spring/5 -> Terminator1/1
  Vehicle Adapter/2(VehSusp) -> Bus Selector1/1

== system TractorTrailer6DOF/Three-Axle Trailer/Vehicle Body ==
  Suspension : Inport
  Hitch : Inport  Port=2
  Bus Selector3 : BusSelector  OutputSignals=Veh.F,Veh.M
  Constant1 : Constant  Value=zeros(3,1)
  Ground : Ground
  Ground1 : Ground
  Selector6 : Selector  InputPortWidth=6  IndexOptions=Index vector (dialog)  Indices=[1 2 3]  OutputSizes=1
  Selector7 : Selector  InputPortWidth=6  IndexOptions=Index vector (dialog)  Indices=[4 5 6]  OutputSizes=1
  Terminator{,1..5} (6 alike) : Terminator
  Trailer Body 6DOF : vehdynlibeom/Trailer Body 6DOF  axleMode=3  extPos=on  extVel=on  extEuler=on  extRotRate=on  htchFMode_f=on  htchMMode_f=on  htchFMode_r=off  htchMMode_r=off  m=trailer.Mass  a=trailer.FrontAxlePositionfromCG  b=trailer.MiddleAxlePositionFromCG  c=trailer.RearAxlePositionfromCG  d=0  h=trailer.HeightCG  dh_f=trailer.HitchDistance  hl_f=0  hh_f=trailer.HitchHeight  dh_r=1  hl_r=0  hh_r=0.1  Xe_o=initialTrailerPosition  xbdot_o=initialTrailerVelocity  eul_o=initialTrailerOrientation  p_o=initialTrailerRotationRates  Iveh=[trailer.RollMomentInertia 0 0; 0 trailer.PitchMomentInertia 0; 0 0 trailer.YawMomentInertia]  w_f=trailer.TrackWidth  w_m=trailer.TrackWidth  w_r=trailer.TrackWidth  z1m=0  z1R=[-.25,.125,.15]  z1I=[1.4,-.2,.1;-.2,1.4,.1;.1,.1,2.25].*0  z2m=0  z2R=[1.4,0,.8]  z2I=[1.4,-.2,.1;-.2,1.4,.1;.1,.1,2.25].*0  z3m=0  z3R=[.75,-.5,.4]  z3I=[5,-.1,-2;-2,9,.1;-.1,.1,6].*0  z4m=0  z4R=[.75,.5,.4]  z4I=[5,-.1,-2;-2,9,.1;-.1,.1,6].*0  z5m=0  z5R=[1.25,-.5,.4]  z5I=[5,-.1,-2;-2,9,.1;-.1,.1,6].*0  z6m=0  z6R=[1.25,-.5,.4]  z6I=[5,-.1,-2;-2,9,.1;-.1,.1,6].*0  z7m=0  z7R=[2,0,.25]  z7I=[1.4,-.2,.1;-.2,1.4,.1;.1,.1,2.25].*0  Af=trailer.FrontalArea  Cd=.3  Cl=.1  Cpm=.1  beta_w=[0:0.01:0.3]  Cs=[0:0.03:0.9]  Cym=[0:0.01:0.3]  Pabs=101325  extTamb=off  Tair=273  g=9.81  xdot_tol=.1  longOff=0  latOff=0  vertOff=0.0112  wrapAng=off  aMode=2
  Vehicle : Outport
  wires:
  Suspension/1 -> Bus Selector3/1
  Selector7/1 -> Trailer Body 6DOF/6
  Trailer Body 6DOF/2 -> Terminator5/1
  Hitch/1 -> Selector7/1, Selector6/1
  Selector6/1 -> Trailer Body 6DOF/5
  Trailer Body 6DOF/7 -> Terminator/1
  Trailer Body 6DOF/3 -> Terminator4/1
  Constant1/1 -> Trailer Body 6DOF/7
  Bus Selector3/2 -> Trailer Body 6DOF/2  "<M>"
  Trailer Body 6DOF/5 -> Terminator2/1
  Ground/1 -> Trailer Body 6DOF/3
  Trailer Body 6DOF/6 -> Terminator1/1
  Trailer Body 6DOF/4 -> Terminator3/1
  Trailer Body 6DOF/1 -> Vehicle/1
  Bus Selector3/1 -> Trailer Body 6DOF/1  "<F>"
  Ground1/1 -> Trailer Body 6DOF/4

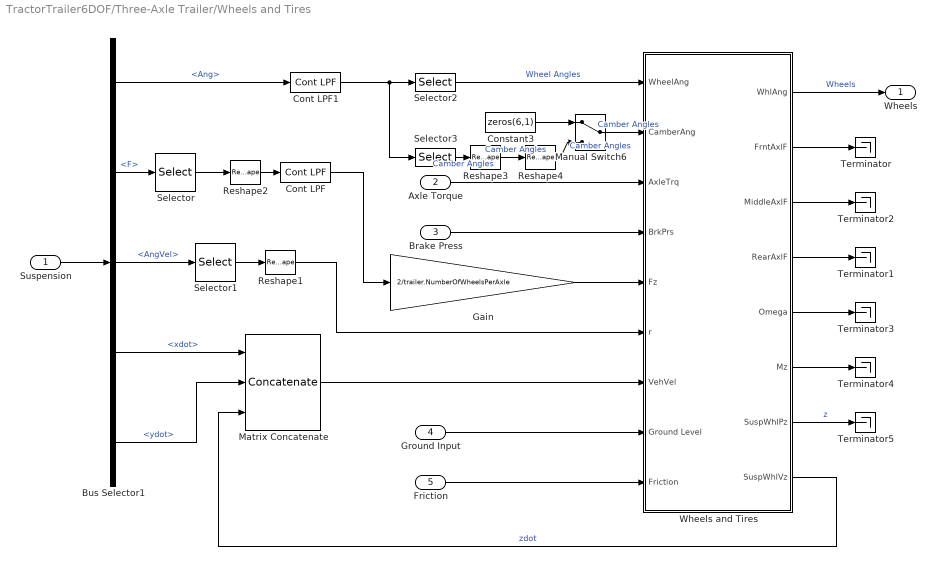
== system TractorTrailer6DOF/Three-Axle Trailer/Wheels and Tires ==
  Suspension : Inport
  Axle Torque : Inport  Port=2
  Brake Press : Inport  Port=3  Unit=Pa
  Ground Input : Inport  Port=4
  Friction : Inport  Port=5
  Bus Selector1 : BusSelector  OutputSignals=Whl.Ang,Whl.F,Whl.AngVel,Whl.xdot,Whl.ydot
  Constant3 : Constant  Value=zeros(6,1)
  Cont LPF : autolibutils/Cont LPF  wc=100*2*pi  AbsoluteTolerance=auto  aMode=2
  Cont LPF1 : autolibutils/Cont LPF  wc=100*2*pi  AbsoluteTolerance=auto  aMode=2
  Gain : Gain  Gain=2/trailer.NumberOfWheelsPerAxle
  Manual Switch6 : ManualSwitch
  Matrix Concatenate : Concatenate  NumInputs=3  Mode=Multidimensional array
  Reshape1 : Reshape
  Reshape2 : Reshape
  Reshape3 : Reshape  OutputDimensionality=Column vector (2-D)
  Reshape4 : Reshape
  Selector : Selector  NumberOfDimensions=2  InputPortWidth=3  IndexOptions=Index vector (dialog),Select all  Indices=[3],1  OutputSizes=1,1
  Selector1 : Selector  NumberOfDimensions=2  InputPortWidth=1  IndexOptions=Index vector (dialog),Select all  Indices=[3],1  OutputSizes=1,1
  Selector2 : Selector  NumberOfDimensions=2  InputPortWidth=3  IndexOptions=Index vector (dialog),Select all  Indices=3,1  OutputSizes=1,1
  Selector3 : Selector  NumberOfDimensions=2  InputPortWidth=3  IndexOptions=Index vector (dialog),Select all  Indices=1,1  OutputSizes=1,1
  Terminator{,1..5} (6 alike) : Terminator
  Wheels and Tires : Subsystem  VariantControl=0
  Wheels : Outport  VectorParamsAs1DForOutWhenUnconnected=off
  wires:
  Wheels and Tires/3(MiddleAxlF) -> Terminator2/1
  Cont LPF1/1 -> Selector2/1, Selector3/1
  Cont LPF/1 -> Gain/1
  Friction/1 -> Wheels and Tires/9(Friction)
  Brake Press/1 -> Wheels and Tires/4(BrkPrs)
  Reshape1/1 -> Wheels and Tires/6(r)
  Bus Selector1/3 -> Selector1/1  "<AngVel>"
  Reshape2/1 -> Cont LPF/1
  Wheels and Tires/7(SuspWhlPz) -> Terminator5/1  "z"
  Bus Selector1/5 -> Matrix Concatenate/2  "<ydot>"
  Bus Selector1/4 -> Matrix Concatenate/1  "<xdot>"
  Suspension/1 -> Bus Selector1/1
  Reshape3/1 -> Reshape4/1  "Camber Angles"
  Bus Selector1/1 -> Cont LPF1/1  "<Ang>"
  Wheels and Tires/8(SuspWhlVz) -> Matrix Concatenate/3  "zdot"
  Ground Input/1 -> Wheels and Tires/8(Ground Level)
  Gain/1 -> Wheels and Tires/5(Fz)
  Selector/1 -> Reshape2/1
  Manual Switch6/1 -> Wheels and Tires/2(CamberAng)  "Camber Angles"
  Constant3/1 -> Manual Switch6/1
  Selector2/1 -> Wheels and Tires/1(WheelAng)  "Wheel Angles"
  Axle Torque/1 -> Wheels and Tires/3(AxleTrq)
  Matrix Concatenate/1 -> Wheels and Tires/7(VehVel)
  Selector1/1 -> Reshape1/1
  Wheels and Tires/6(Mz) -> Terminator4/1
  Wheels and Tires/5(Omega) -> Terminator3/1
  Wheels and Tires/4(RearAxlF) -> Terminator1/1
  Wheels and Tires/2(FrntAxlF) -> Terminator/1
  Bus Selector1/2 -> Selector/1  "<F>"
  Wheels and Tires/1(WhlAng) -> Wheels/1  "Wheels"
  Selector3/1 -> Reshape3/1  "Camber Angles"
  Reshape4/1 -> Manual Switch6/2  "Camber Angles"

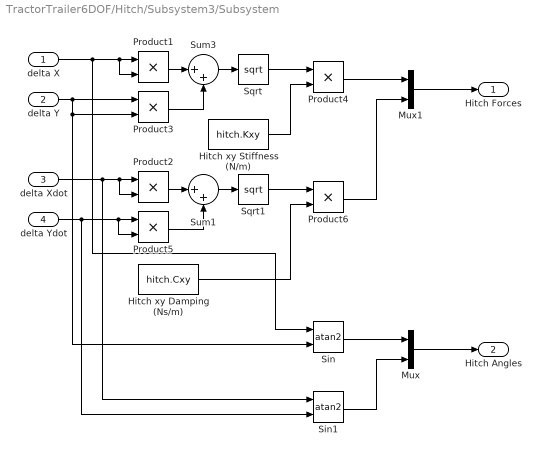
== system TractorTrailer6DOF/Hitch/Subsystem3/Subsystem ==
  delta X : Inport
  delta Y : Inport  Port=2
  delta Xdot : Inport  Port=3
  delta Ydot : Inport  Port=4
  Hitch xy Damping (Ns/m) : Constant  Value=hitch.Cxy
  Hitch xy Stiffness (N/m) : Constant  Value=hitch.Kxy
  Mux : Mux  Inputs=2
  Mux1 : Mux  Inputs=2
  Product{1..6} (6 alike) : Product
  Sin : Trigonometry  Operator=atan2
  Sin1 : Trigonometry  Operator=atan2
  Sqrt : Sqrt
  Sqrt1 : Sqrt
  Sum1 : Sum  Inputs=|++
  Sum3 : Sum  Inputs=|++
  Hitch Forces : Outport
  Hitch Angles : Outport  Port=2
  wires:
  delta Y/1 -> Product3/1, Sin/2, Product3/2
  Sin/1 -> Mux/1
  delta X/1 -> Sin/1, Product1/1, Product1/2
  Sum3/1 -> Sqrt/1
  Product1/1 -> Sum3/1
  Product3/1 -> Sum3/2
  Sqrt/1 -> Product4/1
  Product4/1 -> Mux1/1
  Hitch xy Stiffness (N/m)/1 -> Product4/2
  Sqrt1/1 -> Product6/1
  Product5/1 -> Sum1/2
  Product2/1 -> Sum1/1
  Sum1/1 -> Sqrt1/1
  delta Xdot/1 -> Sin1/1, Product2/2, Product2/1
  Hitch xy Damping (Ns/m)/1 -> Product6/2
  Mux/1 -> Hitch Angles/1
  delta Ydot/1 -> Sin1/2, Product5/1, Product5/2
  Sin1/1 -> Mux/2
  Mux1/1 -> Hitch Forces/1
  Product6/1 -> Mux1/2

== system TractorTrailer6DOF/Hitch/Subsystem3/Subsystem1 ==
  Hitch Forces : Inport
  psi : Inport  Port=2
  Hitch Angles : Inport  Port=3
  Cos : Trigonometry  Operator=cos
  Cos1 : Trigonometry
  Product1 : Product
  Product2 : Product
  Sum : Sum  Inputs=+
  Sum1 : Sum  Inputs=+
  Sum2 : Sum  Inputs=|++
  Fx : Outport
  Fy : Outport  Port=2
  wires:
  Cos1/1 -> Product1/1
  Hitch Angles/1 -> Sum2/1
  Hitch Forces/1 -> Product2/2, Product1/2
  psi/1 -> Sum2/2
  Sum2/1 -> Cos1/1, Cos/1
  Cos/1 -> Product2/1
  Product2/1 -> Sum/1
  Product1/1 -> Sum1/1
  Sum/1 -> Fy/1
  Sum1/1 -> Fx/1

== system TractorTrailer6DOF/Hitch/Subsystem3/Subsystem2 ==
  Hitch Forces : Inport
  psi : Inport  Port=2
  Hitch Angles : Inport  Port=3
  Cos : Trigonometry  Operator=cos
  Cos1 : Trigonometry
  Gain : Gain  Gain=-1
  Product1 : Product
  Product2 : Product
  Sum : Sum  Inputs=+
  Sum1 : Sum  Inputs=+
  Sum2 : Sum  Inputs=|++
  Fx : Outport
  Fy : Outport  Port=2
  wires:
  Product1/1 -> Sum1/1
  Product2/1 -> Sum/1
  Cos/1 -> Product2/1
  Sum2/1 -> Cos/1, Cos1/1
  psi/1 -> Sum2/2
  Hitch Forces/1 -> Gain/1
  Hitch Angles/1 -> Sum2/1
  Cos1/1 -> Product1/1
  Gain/1 -> Product1/2, Product2/2
  Sum/1 -> Fy/1
  Sum1/1 -> Fx/1

== system TractorTrailer6DOF/Hitch/Subsystem3/Subsystem3 ==
  Vehicle Z : Inport
  Trailer Z : Inport  Port=2
  Vehicle Zdot : Inport  Port=3
  Trailer Zdot : Inport  Port=4
  Constant2 : Constant  Value=trailer.HeightCG
  Constant3 : Constant  Value=tractor.HeightCG
  Constant8 : Constant  Value=hitch.F0z
  Gain5 : Gain  Gain=hitch.Kz
  Gain6 : Gain  Gain=hitch.Cz
  Sum1 : Sum  Inputs=|--
  Sum2 : Sum  Inputs=|+-
  Sum3 : Sum  Inputs=|+-
  Sum4 : Sum  Inputs=|+-
  Sum5 : Sum  Inputs=|-+
  Sum6 : Sum  Inputs=|-+
  Trailer Fz : Outport
  wires:
  Vehicle Z/1 -> Sum6/2
  Sum4/1 -> Trailer Fz/1
  Trailer Z/1 -> Sum5/2
  Gain5/1 -> Sum1/1
  Constant8/1 -> Sum4/2
  Sum1/1 -> Sum4/1
  Gain6/1 -> Sum1/2
  Sum2/1 -> Gain5/1
  Trailer Zdot/1 -> Sum3/1
  Vehicle Zdot/1 -> Sum3/2
  Sum3/1 -> Gain6/1
  Constant2/1 -> Sum5/1
  Sum5/1 -> Sum2/1
  Constant3/1 -> Sum6/1
  Sum6/1 -> Sum2/2

== system TractorTrailer6DOF/Hitch/Subsystem3/Trailer Hitch Contact Moment ==
  Vehicle Psi : Inport
  Trailer Psi : Inport  Port=2
  Ground1 : Ground
  Hitch Contact Yaw Moment : Lookup_n-D  NumberOfTableDimensions=1  LookupTableObject=''  BreakpointsForDimension1=[-1 -.9 -45*pi/180 0 45*pi/180 .9 1]  BreakpointsForDimension1FirstPoint=10  BreakpointsForDimension2FirstPoint=10  BreakpointsForDimension1Spacing=12  BreakpointsForDimension2Spacing=12  IndexSearchMethod=Linear search  Table=[-1e6 -1e6 0 0 0 1e6 1e6]  ExtrapMethod=Clip  DiagnosticForOutOfRangeInput=Error  UseLastTableValue=on  InternalRulePriority=Speed  RndMeth=Simplest
  Subtract : Sum  Inputs=+-
  Vector Concatenate1 : Concatenate  NumInputs=3
  Mh : Outport
  wires:
  Trailer Psi/1 -> Subtract/2
  Subtract/1 -> Hitch Contact Yaw Moment/1
  Vehicle Psi/1 -> Subtract/1
  Hitch Contact Yaw Moment/1 -> Vector Concatenate1/3
  Ground1/1 -> Vector Concatenate1/2, Vector Concatenate1/1
  Vector Concatenate1/1 -> Mh/1

== system TractorTrailer6DOF/Three-Axle Tractor/Subsystem1/Driveline ==
  TPowertrain : Inport  PortDimensions=1
  Gear : Inport  Port=2
  AWD : Subsystem  VariantControl=2
  FWD : Subsystem  VariantControl=1
  RWD : Subsystem  VariantControl=0
  TAxles : Outport  PortDimensions=6  VectorParamsAs1DForOutWhenUnconnected=off

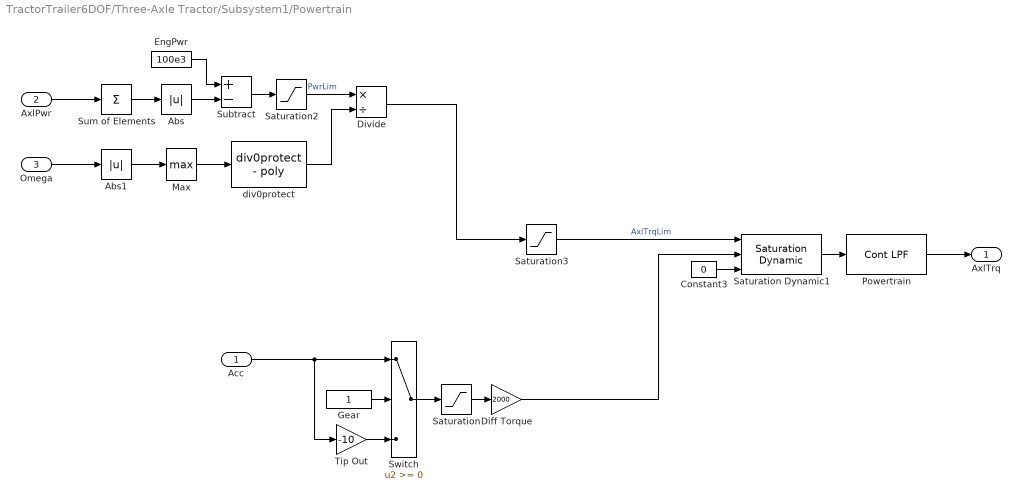
== system TractorTrailer6DOF/Three-Axle Tractor/Subsystem1/Powertrain ==
  Acc : Inport
  AxlPwr : Inport  Port=2  PortDimensions=6
  Omega : Inport  Port=3  PortDimensions=6
  Abs : Abs  ZeroCross=off  SaturateOnIntegerOverflow=off
  Abs1 : Abs  ZeroCross=off  SaturateOnIntegerOverflow=off
  Constant3 : Constant  Value=0
  Diff Torque : Gain  Gain=2000
  Divide : Product  Inputs=*/
  EngPwr : Constant  Value=100e3
  Gear : Constant  SampleTime=-1
  Max : MinMax  Function=max  ZeroCross=off
  Powertrain : autolibutils/Cont LPF  wc=4*pi*2  AbsoluteTolerance=auto  aMode=2
  Saturation : Saturate  UpperLimit=inf  LowerLimit=0  ZeroCross=off
  Saturation Dynamic1 : simulink/Discontinuities/Saturation Dynamic  OutMin=[]  OutMax=[]  OutDataTypeStr=Inherit: Same as second input  OutDataType=fixdt(1, 16)  OutScaling=2^-10  DoSatur=off
  Saturation2 : Saturate  UpperLimit=inf  LowerLimit=100  ZeroCross=off
  Saturation3 : Saturate  UpperLimit=6000  LowerLimit=0  ZeroCross=off
  Subtract : Sum  Inputs=+-
  Sum of Elements : Sum  Inputs=+
  Switch : Switch  ZeroCross=off  SaturateOnIntegerOverflow=off  InputSameDT=off
  Tip Out : Gain  Gain=-10
  div0protect : autolibutils/div0protect - poly  thresh=1  ZeroCross=off  ZeroCross1=on  aMode=2
  AxlTrq : Outport  VectorParamsAs1DForOutWhenUnconnected=off
  wires:
  Abs1/1 -> Max/1
  Max/1 -> div0protect/1
  EngPwr/1 -> Subtract/1
  Saturation2/1 -> Divide/1  "PwrLim"
  Subtract/1 -> Saturation2/1
  div0protect/1 -> Divide/2
  Abs/1 -> Subtract/2
  Sum of Elements/1 -> Abs/1
  Constant3/1 -> Saturation Dynamic1/3
  Tip Out/1 -> Switch/3
  Saturation Dynamic1/1 -> Powertrain/1
  Gear/1 -> Switch/2
  Diff Torque/1 -> Saturation Dynamic1/2
  Saturation/1 -> Diff Torque/1
  Acc/1 -> Switch/1, Tip Out/1
  Switch/1 -> Saturation/1
  Powertrain/1 -> AxlTrq/1
  AxlPwr/1 -> Sum of Elements/1
  Omega/1 -> Abs1/1
  Saturation3/1 -> Saturation Dynamic1/1  "AxlTrqLim"
  Divide/1 -> Saturation3/1

== system TractorTrailer6DOF/Three-Axle Tractor/Vehicle Suspension/Steer Rate Adapter ==
  Veh : Inport
  Add : Sum
  Bus Selector3 : BusSelector  OutputSignals=BdyFrm.Cg.AngVel.r
  Constant : Constant  Value=zeros(1,6)
  Matrix Concatenate : Concatenate  NumInputs=3  Mode=Multidimensional array
  Matrix Concatenate1 : Concatenate  NumInputs=3  Mode=Multidimensional array
  Mux : Mux  Inputs=6
  Reshape2 : Reshape  OutputDimensionality=Row vector (2-D)
  Reshape3 : Reshape  OutputDimensionality=Row vector (2-D)
  Reshape4 : Reshape  OutputDimensionality=Row vector (2-D)
  SteerRates : Constant  Value=zeros(1,6)
  AngVel : Outport  VectorParamsAs1DForOutWhenUnconnected=off
  wires:
  Reshape2/1 -> Matrix Concatenate1/1, Matrix Concatenate1/3, Matrix Concatenate1/2
  Constant/1 -> Reshape3/1
  Mux/1 -> Reshape4/1
  Bus Selector3/1 -> Mux/2, Mux/4, Mux/5, Mux/6, Mux/3, Mux/1  "<r>"
  Matrix Concatenate/1 -> Add/2
  SteerRates/1 -> Reshape2/1
  Reshape4/1 -> Matrix Concatenate/3
  Reshape3/1 -> Matrix Concatenate/2, Matrix Concatenate/1
  Matrix Concatenate1/1 -> Add/1
  Veh/1 -> Bus Selector3/1
  Add/1 -> AngVel/1  "AngVel"

== system TractorTrailer6DOF/Three-Axle Tractor/Vehicle Suspension/Steering Adapter ==
  Steer : Inport
  Reshape1 : Reshape  OutputDimensionality=Row vector (2-D)
  StrgAng : Outport  VectorParamsAs1DForOutWhenUnconnected=off
  wires:
  Reshape1/1 -> StrgAng/1
  Steer/1 -> Reshape1/1

== system TractorTrailer6DOF/Three-Axle Tractor/Vehicle Suspension/Vehicle Adapter ==
  Veh : Inport
  Bus Creator3 : BusCreator  Inputs=2
  Bus Selector1 : BusSelector  OutputSignals=InertFrm.FrntAxl.Lft.Disp.X,InertFrm.FrntAxl.Lft.Disp.Y,InertFrm.FrntAxl.Lft.Disp.Z,InertFrm.FrntAxl.Rght.Disp.X,InertFrm.FrntAxl.Rght.Disp.Y,InertFrm.FrntAxl.Rght.Disp.Z,InertFrm.MidlAxl.Lft.Disp.X,InertFrm.MidlAxl.Lft.Disp.Y,InertFrm.MidlAxl.Lft.Disp.Z,InertFrm.MidlAxl.Rght.Disp.X,InertFrm.MidlAxl.Rght.Disp.Y,InertFrm.MidlAxl.Rght.Disp.Z,InertFrm.RearAxl.Lft.Disp.X,InertFrm.RearAxl.Lft.Disp.Y,InertFrm.RearAxl.Lft.Disp.Z,InertFrm.RearAxl.Rght.Disp.X,InertFrm.RearAxl.Rght.Disp.Y,InertFrm.RearAxl.Rght.Disp.Z
  Bus Selector2 : BusSelector  OutputSignals=BdyFrm.FrntAxl.Lft.Vel.xdot,BdyFrm.FrntAxl.Lft.Vel.ydot,BdyFrm.FrntAxl.Lft.Vel.zdot,BdyFrm.FrntAxl.Rght.Vel.xdot,BdyFrm.FrntAxl.Rght.Vel.ydot,BdyFrm.FrntAxl.Rght.Vel.zdot,BdyFrm.MidlAxl.Lft.Vel.xdot,BdyFrm.MidlAxl.Lft.Vel.ydot,BdyFrm.MidlAxl.Lft.Vel.zdot,BdyFrm.MidlAxl.Rght.Vel.xdot,BdyFrm.MidlAxl.Rght.Vel.ydot,BdyFrm.MidlAxl.Rght.Vel.zdot,BdyFrm.RearAxl.Lft.Vel.xdot,BdyFrm.RearAxl.Lft.Vel.ydot,BdyFrm.RearAxl.Lft.Vel.zdot,BdyFrm.RearAxl.Rght.Vel.xdot,BdyFrm.RearAxl.Rght.Vel.ydot,BdyFrm.RearAxl.Rght.Vel.zdot
  Bus Selector3 : BusSelector  OutputSignals=InertFrm.FrntAxl.Lft.Vel.Xdot,InertFrm.FrntAxl.Lft.Vel.Ydot,InertFrm.FrntAxl.Lft.Vel.Zdot,InertFrm.FrntAxl.Rght.Vel.Xdot,InertFrm.FrntAxl.Rght.Vel.Ydot,InertFrm.FrntAxl.Rght.Vel.Zdot,InertFrm.MidlAxl.Lft.Vel.Xdot,InertFrm.MidlAxl.Lft.Vel.Ydot,InertFrm.MidlAxl.Lft.Vel.Zdot,InertFrm.MidlAxl.Rght.Vel.Xdot,InertFrm.MidlAxl.Rght.Vel.Ydot,InertFrm.MidlAxl.Rght.Vel.Zdot,InertFrm.RearAxl.Lft.Vel.Xdot,InertFrm.RearAxl.Lft.Vel.Ydot,InertFrm.RearAxl.Lft.Vel.Zdot,InertFrm.RearAxl.Rght.Vel.Xdot,InertFrm.RearAxl.Rght.Vel.Ydot,InertFrm.RearAxl.Rght.Vel.Zdot
  Inertial Frame CG to Axle Offset : Constant  Value=[zeros(2,6);tractor.HeightCG*ones(1,6)]
  Mux1 : Mux  Inputs=18
  Mux2 : Mux  Inputs=18
  Mux3 : Mux  Inputs=18
  Reshape : Reshape  OutputDimensionality=Customize  OutputDimensions=[3,6]
  Reshape1 : Reshape  OutputDimensionality=Customize  OutputDimensions=[3,6]
  Reshape2 : Reshape  OutputDimensionality=Customize  OutputDimensions=[3,6]
  Sum : Sum  Inputs=|+-
  VehSusp : Outport  VectorParamsAs1DForOutWhenUnconnected=off
  VehVBody : Outport  Port=2  VectorParamsAs1DForOutWhenUnconnected=off
  wires:
  Veh/1 -> Bus Selector2/1, Bus Selector3/1, Bus Selector1/1
  Reshape2/1 -> VehVBody/1  "V"
  Bus Creator3/1 -> VehSusp/1  "Veh"
  Reshape/1 -> Sum/1
  Mux1/1 -> Reshape2/1
  Mux2/1 -> Reshape/1
  Inertial Frame CG to Axle Offset/1 -> Sum/2
  Sum/1 -> Bus Creator3/1  "P"
  Bus Selector1/1 -> Mux2/1  "<X>"
  Bus Selector1/2 -> Mux2/2  "<Y>"
  Bus Selector1/3 -> Mux2/3  "<Z>"
  Bus Selector1/4 -> Mux2/4  "<X>"
  Bus Selector1/5 -> Mux2/5  "<Y>"
  Bus Selector1/6 -> Mux2/6  "<Z>"
  Bus Selector1/7 -> Mux2/7  "<X>"
  Bus Selector1/8 -> Mux2/8  "<Y>"
  Bus Selector1/9 -> Mux2/9  "<Z>"
  Bus Selector1/10 -> Mux2/10  "<X>"
  Bus Selector1/11 -> Mux2/11  "<Y>"
  Bus Selector1/12 -> Mux2/12  "<Z>"
  Bus Selector1/13 -> Mux2/13  "<X>"
  Bus Selector1/14 -> Mux2/14  "<Y>"
  Bus Selector1/15 -> Mux2/15  "<Z>"
  Bus Selector1/16 -> Mux2/16  "<X>"
  Bus Selector1/17 -> Mux2/17  "<Y>"
  Bus Selector1/18 -> Mux2/18  "<Z>"
  Bus Selector2/1 -> Mux1/1  "<xdot>"
  Bus Selector2/2 -> Mux1/2  "<ydot>"
  Bus Selector2/3 -> Mux1/3  "<zdot>"
  Bus Selector2/4 -> Mux1/4  "<xdot>"
  Bus Selector2/5 -> Mux1/5  "<ydot>"
  Bus Selector2/6 -> Mux1/6  "<zdot>"
  Bus Selector2/7 -> Mux1/7  "<xdot>"
  Bus Selector2/8 -> Mux1/8  "<ydot>"
  Bus Selector2/9 -> Mux1/9  "<zdot>"
  Bus Selector2/10 -> Mux1/10  "<xdot>"
  Bus Selector2/11 -> Mux1/11  "<ydot>"
  Bus Selector2/12 -> Mux1/12  "<zdot>"
  Bus Selector2/13 -> Mux1/13  "<xdot>"
  Bus Selector2/14 -> Mux1/14  "<ydot>"
  Bus Selector2/15 -> Mux1/15  "<zdot>"
  Bus Selector2/16 -> Mux1/16  "<xdot>"
  Bus Selector2/17 -> Mux1/17  "<ydot>"
  Bus Selector2/18 -> Mux1/18  "<zdot>"
  Bus Selector3/2 -> Mux3/2  "<Ydot>"
  Mux3/1 -> Reshape1/1
  Bus Selector3/13 -> Mux3/13  "<Xdot>"
  Bus Selector3/14 -> Mux3/14  "<Ydot>"
  Bus Selector3/12 -> Mux3/12  "<Zdot>"
  Bus Selector3/9 -> Mux3/9  "<Zdot>"
  Bus Selector3/10 -> Mux3/10  "<Xdot>"
  Bus Selector3/7 -> Mux3/7  "<Xdot>"
  Bus Selector3/17 -> Mux3/17  "<Ydot>"
  Bus Selector3/5 -> Mux3/5  "<Ydot>"
  Bus Selector3/3 -> Mux3/3  "<Zdot>"
  Bus Selector3/15 -> Mux3/15  "<Zdot>"
  Bus Selector3/6 -> Mux3/6  "<Zdot>"
  Bus Selector3/8 -> Mux3/8  "<Ydot>"
  Bus Selector3/1 -> Mux3/1  "<Xdot>"
  Reshape1/1 -> Bus Creator3/2  "V"
  Bus Selector3/16 -> Mux3/16  "<Xdot>"
  Bus Selector3/4 -> Mux3/4  "<Xdot>"
  Bus Selector3/11 -> Mux3/11  "<Ydot>"
  Bus Selector3/18 -> Mux3/18  "<Zdot>"

== system TractorTrailer6DOF/Three-Axle Tractor/Vehicle Suspension/Wheel  Adapter ==
  Wheels : Inport
  Bus Selector : BusSelector  OutputSignals=TireFrame.Fx,TireFrame.Fy
  Bus Selector1 : BusSelector  OutputSignals=TireFrame.Re
  Bus Selector2 : BusSelector  OutputSignals=TireFrame.Mx,TireFrame.My,TireFrame.Mz
  Bus Selector3 : BusSelector  OutputSignals=TireFrame.z,TireFrame.zdot
  Matrix Concatenate : Concatenate  NumInputs=3  Mode=Multidimensional array
  Reshape{,1..7} (8 alike) : Reshape  OutputDimensionality=Row vector (2-D)
  WhlFx : Outport  VectorParamsAs1DForOutWhenUnconnected=off
  WhlFy : Outport  Port=2  VectorParamsAs1DForOutWhenUnconnected=off
  z : Outport  Port=3  VectorParamsAs1DForOutWhenUnconnected=off
  zdot : Outport  Port=4  VectorParamsAs1DForOutWhenUnconnected=off
  M : Outport  Port=5  VectorParamsAs1DForOutWhenUnconnected=off
  Re : Outport  Port=6  VectorParamsAs1DForOutWhenUnconnected=off
  wires:
  Reshape7/1 -> WhlFy/1
  Reshape6/1 -> WhlFx/1
  Bus Selector/1 -> Reshape6/1  "<Fx>"
  Bus Selector/2 -> Reshape7/1  "<Fy>"
  Bus Selector3/1 -> Reshape/1  "<z>"
  Wheels/1 -> Bus Selector1/1, Bus Selector2/1, Bus Selector3/1, Bus Selector/1
  Bus Selector3/2 -> Reshape2/1  "<zdot>"
  Reshape2/1 -> zdot/1  "zdot"
  Bus Selector1/1 -> Reshape1/1  "<Re>"
  Reshape1/1 -> Re/1  "Re"
  Bus Selector2/1 -> Reshape3/1  "<Mx>"
  Bus Selector2/2 -> Reshape4/1  "<My>"
  Bus Selector2/3 -> Reshape5/1  "<Mz>"
  Reshape3/1 -> Matrix Concatenate/1
  Reshape4/1 -> Matrix Concatenate/2
  Reshape5/1 -> Matrix Concatenate/3
  Matrix Concatenate/1 -> M/1  "M"
  Reshape/1 -> z/1  "z"
